simulink model "Quadrotor"  (Simulink 10.2)
settings: Solver=ode1  StartTime=0.0  StopTime=10  FixedStep=1e-4  RelTol=1e-3
settings Model: Creator=贺嘉辣  LastModifiedBy=贺嘉辣
settings DataIOCC: SaveFormat=Dataset  SignalLoggingSaveFormat=Dataset  ReturnWorkspaceOutputs=on
settings OptimizationCC: LifeSpan=auto
settings DebuggingCC: UnderspecifiedInitializationDetection=Simplified  MergeDetectMultiDrivingBlocksExec=error  FcnCallInpInsideContextMsg=error  SFUnexpectedBacktrackingDiag=error  SFNoUnconditionalDefaultTransitionDiag=error  SFExecutionAtInitializationDiag=warning  ArithmeticOperatorsInVariantConditions=error
settings HardwareCC: ProdBitPerPointer=64  ProdBitPerSizeT=64  ProdBitPerPtrDiffT=64  ProdLargestAtomicFloat=Float  ProdIntDivRoundTo=Zero  ProdEndianess=LittleEndian  ProdWordSize=64  ProdHWDeviceType=Intel->x86-64 (Windows64)
settings ModelReferenceCC: PropagateSignalLabelsOutOfModel=on
settings SFSimCC: SimUseLocalCustomCode=on  CustomCodeUndefinedFunction=FilterOut
settings RTWCC: RTWUseLocalCustomCode=on
settings CodeAppCC: StateflowObjectComments=off
settings GRTTargetCC: TargetLangStandard=C99 (ISO)  CombineOutputUpdateFcns=on  GRTInterface=off
settings ConfigComp: CovMetricSettings=dwe  CovSaveCumulativeToWorkspaceVar=off  CovSaveSingleToWorkspaceVar=off  CovExternalEMLEnable=on

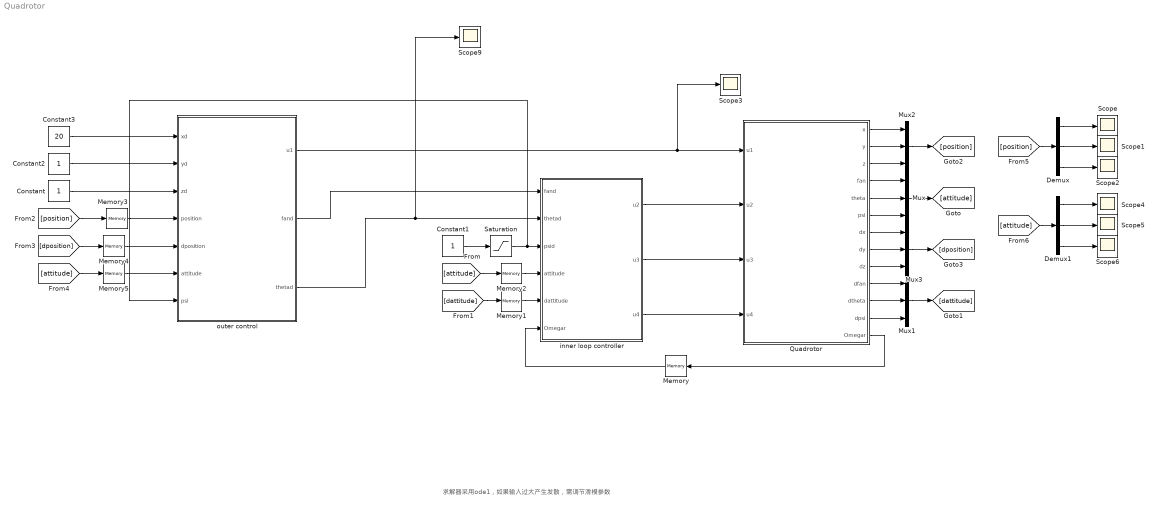
== system Quadrotor ==
  note: 求解器采用ode1，如果输入过大产生发散，需调节滑模参数
  Constant : Constant
  Constant1 : Constant
  Constant2 : Constant
  Constant3 : Constant  Value=20
  Demux : Demux  Outputs=3
  Demux1 : Demux  Outputs=3
  Memory{,1..5} (6 alike) : Memory
  Mux{,1..3} (4 alike) : Mux  Inputs=[1 1 1]
  Quadrotor : Subsystem  mask{m=0.65, g=9.8, Ixx=7.5e-3, Iyy=7.5e-3, Izz=1.3e-2, L=0.23, rho=3.1e-5, gama=7.5e-7, Ir=6e-5}
      mask prompts: m "无人机质量"; g "重力加速度"; Ixx "四旋翼绕X轴转动惯量"; Iyy "四旋翼绕Y轴转动惯量"; Izz "四旋翼绕Z轴转动惯量"; L "四旋翼臂长"; rho "四旋翼升力系数"; gama "空气阻力系数"; Ir "四旋翼转子转动惯量"
  Saturation : Saturate  UpperLimit=pi  LowerLimit=-pi
  Scope{,1..6,9} (8 alike) : Scope
  inner loop controller : Subsystem  mask{Ir=6e-5, Ixx=7.5e-3, Iyy=7.5e-3, Izz=1.3e-2}
      mask prompts: Ir "无人机转子惯量"; Ixx "无人机绕x轴转动惯量"; Iyy "无人机绕y轴转动惯量"; Izz "无人机绕z轴转动惯量"
  outer control : Subsystem  mask{m=0.65, g=9.8}
      mask prompts: m "无人机质量"; g "重力加速度"
  wires:
  inner loop controller/1(u2) -> Quadrotor/2(u2)
  inner loop controller/2(u3) -> Quadrotor/3(u3)
  Quadrotor/4(fan) -> Mux/1
  Quadrotor/5(theta) -> Mux/2
  Quadrotor/6(psi) -> Mux/3
  Mux/1 -> [attitude]
  Quadrotor/10(dfan) -> Mux1/1
  Quadrotor/11(dtheta) -> Mux1/2
  Quadrotor/12(dpsi) -> Mux1/3
  Mux1/1 -> [dattitude]
  [dattitude] -> Memory1/1
  [attitude] -> Memory2/1
  Quadrotor/13(Omegar) -> Memory/1
  Quadrotor/1(x) -> Mux2/1
  Quadrotor/2(y) -> Mux2/2
  Quadrotor/3(z) -> Mux2/3
  Mux2/1 -> [position]
  Memory/1 -> inner loop controller/6(Omegar)
  Memory1/1 -> inner loop controller/5(dattitude)
  Memory2/1 -> inner loop controller/4(attitude)
  Quadrotor/7(dx) -> Mux3/1
  Quadrotor/8(dy) -> Mux3/2
  Quadrotor/9(dz) -> Mux3/3
  Mux3/1 -> [dposition]
  [position] -> Memory3/1
  [dposition] -> Memory4/1
  Memory3/1 -> outer control/4(position)
  Memory4/1 -> outer control/5(dposition)
  [attitude] -> Memory5/1
  Memory5/1 -> outer control/6(attitude)
  Constant/1 -> outer control/3(zd)
  Constant1/1 -> Saturation/1
  Constant2/1 -> outer control/2(yd)
  Constant3/1 -> outer control/1(xd)
  inner loop controller/3(u4) -> Quadrotor/4(u4)
  outer control/2(fand) -> inner loop controller/1(fand)
  outer control/3(thetad) -> Scope9/1, inner loop controller/2(thetad)
  outer control/1(u1) -> Scope3/1, Quadrotor/1(u1)
  Saturation/1 -> outer control/7(psi), inner loop controller/3(psid)
  [position] -> Demux/1
  Demux/1 -> Scope/1
  Demux/2 -> Scope1/1
  Demux/3 -> Scope2/1
  [attitude] -> Demux1/1
  Demux1/3 -> Scope6/1
  Demux1/2 -> Scope5/1
  Demux1/1 -> Scope4/1

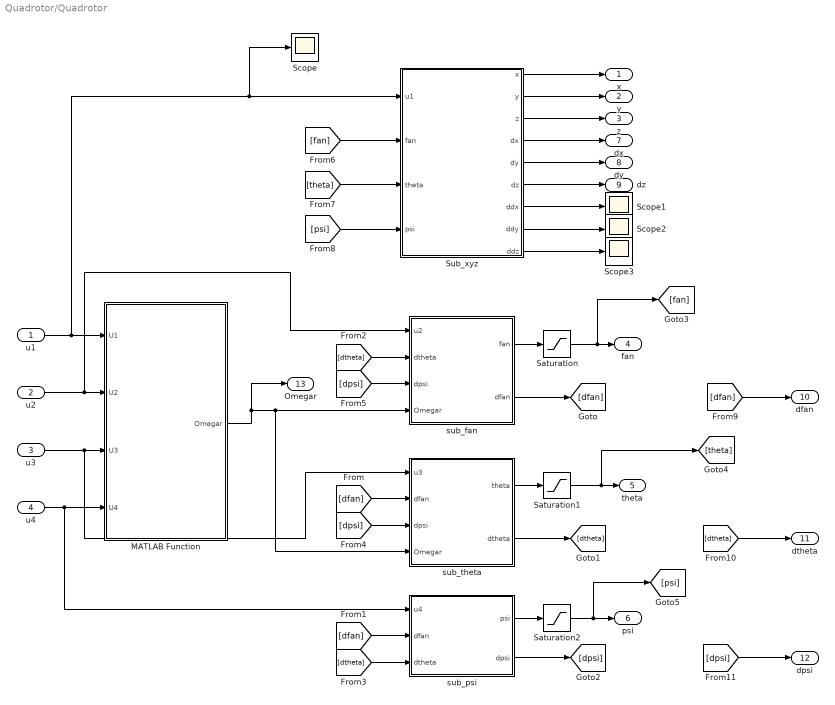
== system Quadrotor/Quadrotor ==
  u1 : Inport
  u2 : Inport  Port=2
  u3 : Inport  Port=3
  u4 : Inport  Port=4
  MATLAB Function : MATLAB Function  TreatAsAtomicUnit=on
  Saturation : Saturate  UpperLimit=pi/2  LowerLimit=-pi/2
  Saturation1 : Saturate  UpperLimit=pi/2  LowerLimit=-pi/2
  Saturation2 : Saturate  UpperLimit=pi  LowerLimit=-pi
  Scope{,1..3} (4 alike) : Scope
  Sub_xyz : Subsystem
  sub_fan : Subsystem
  sub_psi : Subsystem
  sub_theta : Subsystem
  x : Outport
  y : Outport  Port=2
  z : Outport  Port=3
  fan : Outport  Port=4
  theta : Outport  Port=5
  psi : Outport  Port=6
  dx : Outport  Port=7
  dy : Outport  Port=8
  dz : Outport  Port=9
  dfan : Outport  Port=10
  dtheta : Outport  Port=11
  dpsi : Outport  Port=12
  Omegar : Outport  Port=13
  wires:
  u2/1 -> sub_fan/1(u2), MATLAB Function/2(U2)
  u3/1 -> sub_theta/1(u3), MATLAB Function/3(U3)
  u4/1 -> sub_psi/1(u4), MATLAB Function/4(U4)
  sub_fan/1(fan) -> Saturation/1
  sub_theta/1(theta) -> Saturation1/1
  sub_psi/1(psi) -> Saturation2/1
  sub_fan/2(dfan) -> [dfan]
  [dfan] -> sub_theta/2(dfan)
  [dfan] -> sub_psi/2(dfan)
  sub_theta/2(dtheta) -> [dtheta]
  sub_psi/2(dpsi) -> [dpsi]
  [dtheta] -> sub_fan/2(dtheta)
  [dtheta] -> sub_psi/3(dtheta)
  [dpsi] -> sub_theta/3(dpsi)
  [dpsi] -> sub_fan/3(dpsi)
  u1/1 -> Scope/1, Sub_xyz/1(u1), MATLAB Function/1(U1)
  Sub_xyz/1(x) -> x/1
  Sub_xyz/2(y) -> y/1
  Sub_xyz/3(z) -> z/1
  [fan] -> Sub_xyz/2(fan)
  [theta] -> Sub_xyz/3(theta)
  [psi] -> Sub_xyz/4(psi)
  MATLAB Function/1(Omegar) -> Omegar/1, sub_theta/4(Omegar), sub_fan/4(Omegar)
  Sub_xyz/4(dx) -> dx/1
  Sub_xyz/5(dy) -> dy/1
  Sub_xyz/6(dz) -> dz/1
  [dfan] -> dfan/1
  [dtheta] -> dtheta/1
  [dpsi] -> dpsi/1
  Saturation/1 -> fan/1, [fan]
  Saturation1/1 -> theta/1, [theta]
  Saturation2/1 -> psi/1, [psi]
  Sub_xyz/7(ddx) -> Scope1/1
  Sub_xyz/8(ddy) -> Scope2/1
  Sub_xyz/9(ddz) -> Scope3/1

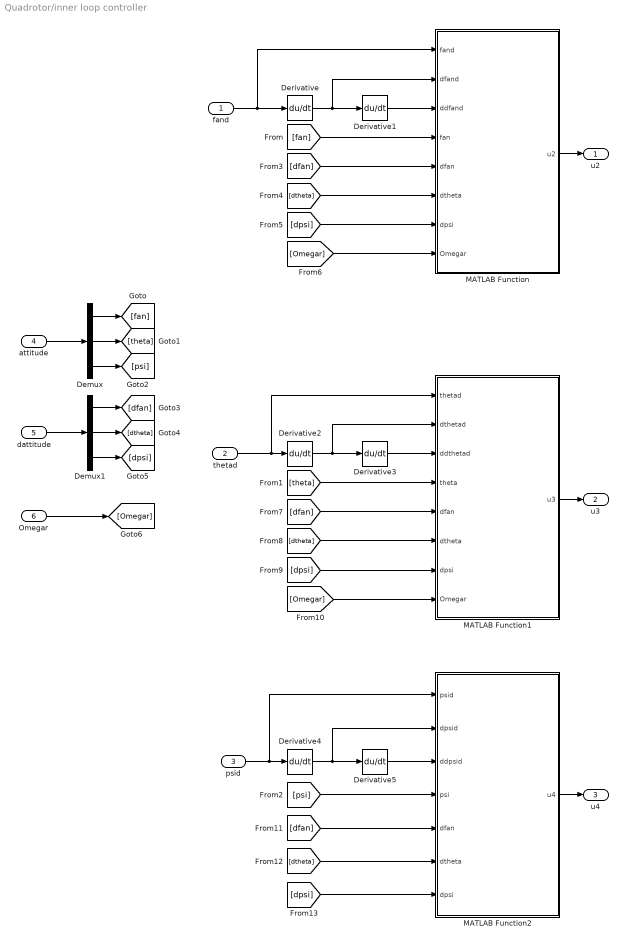
== system Quadrotor/inner loop controller ==
  fand : Inport
  thetad : Inport  Port=2
  psid : Inport  Port=3
  attitude : Inport  Port=4
  dattitude : Inport  Port=5
  Omegar : Inport  Port=6
  Demux : Demux  Outputs=[1 1 1]
  Demux1 : Demux  Outputs=[1 1 1]
  Derivative{,1..5} (6 alike) : Derivative
  MATLAB Function : MATLAB Function  TreatAsAtomicUnit=on
  MATLAB Function1 : MATLAB Function  TreatAsAtomicUnit=on
  MATLAB Function2 : MATLAB Function  TreatAsAtomicUnit=on
  u2 : Outport
  u3 : Outport  Port=2
  u4 : Outport  Port=3
  wires:
  fand/1 -> MATLAB Function/1(fand), Derivative/1
  Derivative/1 -> MATLAB Function/2(dfand), Derivative1/1
  Derivative1/1 -> MATLAB Function/3(ddfand)
  MATLAB Function/1(u2) -> u2/1
  attitude/1 -> Demux/1
  Demux/1 -> [fan]
  Demux/2 -> [theta]
  Demux/3 -> [psi]
  [fan] -> MATLAB Function/4(fan)
  dattitude/1 -> Demux1/1
  Demux1/3 -> [dpsi]
  Demux1/2 -> [dtheta]
  Demux1/1 -> [dfan]
  [dfan] -> MATLAB Function/5(dfan)
  [dtheta] -> MATLAB Function/6(dtheta)
  [dpsi] -> MATLAB Function/7(dpsi)
  Omegar/1 -> [Omegar]
  [Omegar] -> MATLAB Function/8(Omegar)
  Derivative2/1 -> MATLAB Function1/2(dthetad), Derivative3/1
  thetad/1 -> MATLAB Function1/1(thetad), Derivative2/1
  Derivative3/1 -> MATLAB Function1/3(ddthetad)
  MATLAB Function1/1(u3) -> u3/1
  [theta] -> MATLAB Function1/4(theta)
  [dfan] -> MATLAB Function1/5(dfan)
  [dtheta] -> MATLAB Function1/6(dtheta)
  [dpsi] -> MATLAB Function1/7(dpsi)
  [Omegar] -> MATLAB Function1/8(Omegar)
  Derivative4/1 -> MATLAB Function2/2(dpsid), Derivative5/1
  Derivative5/1 -> MATLAB Function2/3(ddpsid)
  psid/1 -> MATLAB Function2/1(psid), Derivative4/1
  [psi] -> MATLAB Function2/4(psi)
  [dpsi] -> MATLAB Function2/7(dpsi)
  [dtheta] -> MATLAB Function2/6(dtheta)
  [dfan] -> MATLAB Function2/5(dfan)
  MATLAB Function2/1(u4) -> u4/1

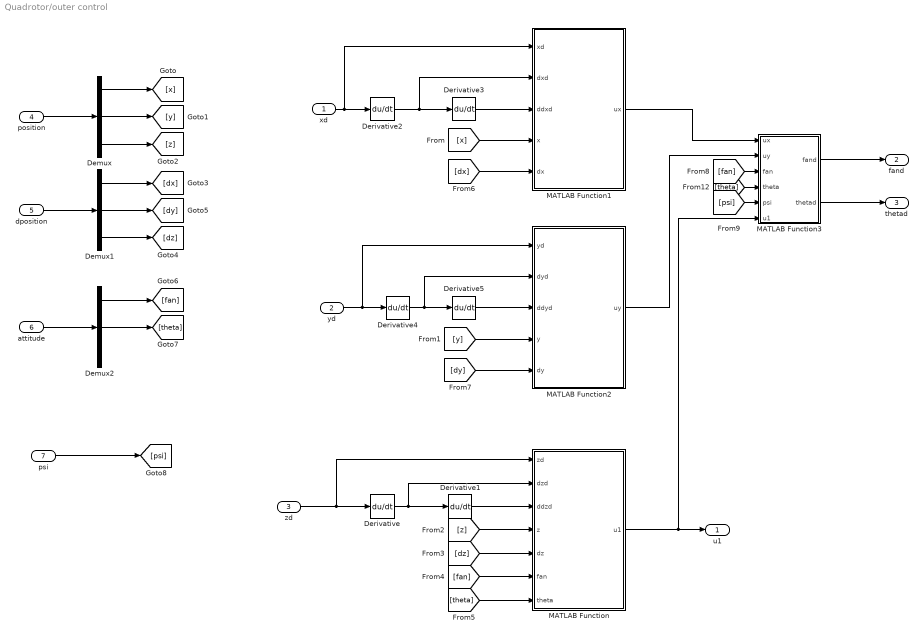
== system Quadrotor/outer control ==
  xd : Inport
  yd : Inport  Port=2
  zd : Inport  Port=3
  position : Inport  Port=4
  dposition : Inport  Port=5
  attitude : Inport  Port=6
  psi : Inport  Port=7
  Demux : Demux  Outputs=[1 1 1]
  Demux1 : Demux  Outputs=[1 1 1]
  Demux2 : Demux  Outputs=[1 1 1]
  Derivative{,1..5} (6 alike) : Derivative
  MATLAB Function : MATLAB Function  TreatAsAtomicUnit=on
  MATLAB Function1 : MATLAB Function  TreatAsAtomicUnit=on
  MATLAB Function2 : MATLAB Function  TreatAsAtomicUnit=on
  MATLAB Function3 : MATLAB Function  TreatAsAtomicUnit=on
  u1 : Outport
  fand : Outport  Port=2
  thetad : Outport  Port=3
  wires:
  zd/1 -> MATLAB Function/1(zd), Derivative/1
  Derivative/1 -> MATLAB Function/2(dzd), Derivative1/1
  position/1 -> Demux/1
  dposition/1 -> Demux1/1
  Demux/1 -> [x]
  Demux/2 -> [y]
  Demux/3 -> [z]
  Demux1/1 -> [dx]
  Demux1/3 -> [dz]
  Demux1/2 -> [dy]
  [z] -> MATLAB Function/4(z)
  [dz] -> MATLAB Function/5(dz)
  attitude/1 -> Demux2/1
  Demux2/1 -> [fan]
  Demux2/2 -> [theta]
  [fan] -> MATLAB Function/6(fan)
  [theta] -> MATLAB Function/7(theta)
  MATLAB Function/1(u1) -> MATLAB Function3/6(u1), u1/1
  Derivative2/1 -> MATLAB Function1/2(dxd), Derivative3/1
  xd/1 -> MATLAB Function1/1(xd), Derivative2/1
  [x] -> MATLAB Function1/4(x)
  [dx] -> MATLAB Function1/5(dx)
  yd/1 -> MATLAB Function2/1(yd), Derivative4/1
  Derivative4/1 -> MATLAB Function2/2(dyd), Derivative5/1
  [dy] -> MATLAB Function2/5(dy)
  [y] -> MATLAB Function2/4(y)
  MATLAB Function1/1(ux) -> MATLAB Function3/1(ux)
  MATLAB Function2/1(uy) -> MATLAB Function3/2(uy)
  [psi] -> MATLAB Function3/5(psi)
  MATLAB Function3/1(fand) -> fand/1
  MATLAB Function3/2(thetad) -> thetad/1
  [theta] -> MATLAB Function3/4(theta)
  [fan] -> MATLAB Function3/3(fan)
  Derivative3/1 -> MATLAB Function1/3(ddxd)
  Derivative5/1 -> MATLAB Function2/3(ddyd)
  Derivative1/1 -> MATLAB Function/3(ddzd)
  psi/1 -> [psi]

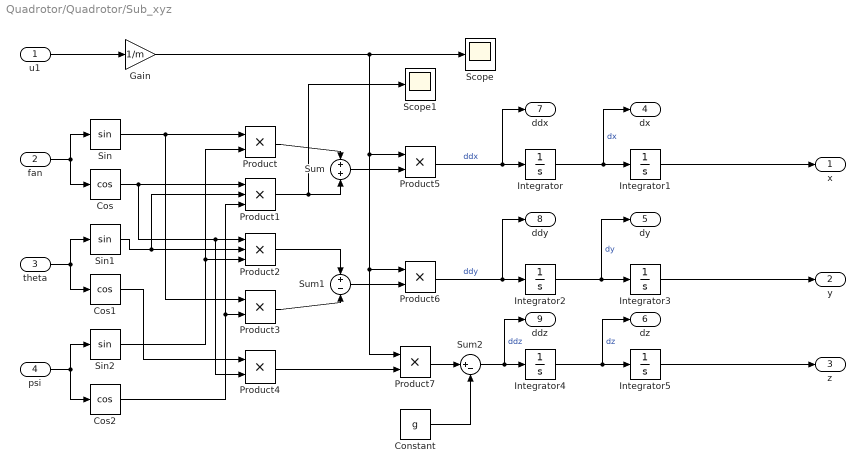
== system Quadrotor/Quadrotor/Sub_xyz ==
  u1 : Inport
  fan : Inport  Port=2
  theta : Inport  Port=3
  psi : Inport  Port=4
  Constant : Constant  Value=g
  Cos : Trigonometry  Operator=cos
  Cos1 : Trigonometry  Operator=cos
  Cos2 : Trigonometry  Operator=cos
  Gain : Gain  Gain=1/m
  Integrator{,1..5} (6 alike) : Integrator
  Product{,3..7} (6 alike) : Product
  Product1 : Product  Inputs=3
  Product2 : Product  Inputs=3
  Scope : Scope
  Scope1 : Scope
  Sin : Trigonometry
  Sin1 : Trigonometry
  Sin2 : Trigonometry
  Sum : Sum  Inputs=+|+
  Sum1 : Sum  Inputs=+|-
  Sum2 : Sum  Inputs=|+-
  x : Outport
  y : Outport  Port=2
  z : Outport  Port=3
  dx : Outport  Port=4
  dy : Outport  Port=5
  dz : Outport  Port=6
  ddx : Outport  Port=7
  ddy : Outport  Port=8
  ddz : Outport  Port=9
  wires:
  u1/1 -> Gain/1
  fan/1 -> Cos/1, Sin/1
  theta/1 -> Cos1/1, Sin1/1
  psi/1 -> Cos2/1, Sin2/1
  Sin/1 -> Product3/1, Product/1
  Sin2/1 -> Product/2, Product2/3
  Cos/1 -> Product4/2, Product2/1, Product1/1
  Sin1/1 -> Product2/2, Product1/2
  Cos2/1 -> Product1/3, Product3/2
  Product/1 -> Sum/1
  Product1/1 -> Scope1/1, Sum/2
  Cos1/1 -> Product4/1
  Product2/1 -> Sum1/1
  Product3/1 -> Sum1/2
  Sum/1 -> Product5/2
  Sum1/1 -> Product6/2
  Product4/1 -> Product7/2
  Gain/1 -> Scope/1, Product7/1, Product6/1, Product5/1
  Product5/1 -> ddx/1, Integrator/1  "ddx"
  Integrator/1 -> dx/1, Integrator1/1  "dx"
  Product6/1 -> ddy/1, Integrator2/1  "ddy"
  Integrator2/1 -> dy/1, Integrator3/1  "dy"
  Product7/1 -> Sum2/1
  Constant/1 -> Sum2/2
  Sum2/1 -> ddz/1, Integrator4/1  "ddz"
  Integrator4/1 -> dz/1, Integrator5/1  "dz"
  Integrator3/1 -> y/1
  Integrator1/1 -> x/1
  Integrator5/1 -> z/1

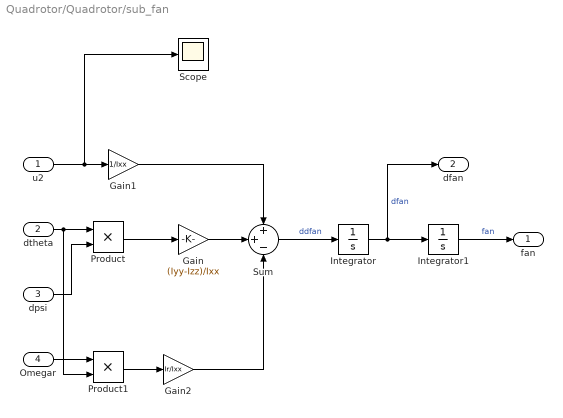
== system Quadrotor/Quadrotor/sub_fan ==
  u2 : Inport
  dtheta : Inport  Port=2
  dpsi : Inport  Port=3
  Omegar : Inport  Port=4
  Gain : Gain  Gain=(Iyy-Izz)/Ixx
  Gain1 : Gain  Gain=1/Ixx
  Gain2 : Gain  Gain=Ir/Ixx
  Integrator : Integrator
  Integrator1 : Integrator
  Product : Product
  Product1 : Product
  Scope : Scope
  Sum : Sum  Inputs=++-
  fan : Outport
  dfan : Outport  Port=2
  wires:
  Sum/1 -> Integrator/1  "ddfan"
  Integrator/1 -> dfan/1, Integrator1/1  "dfan"
  Integrator1/1 -> fan/1  "fan"
  dtheta/1 -> Product1/2, Product/1
  dpsi/1 -> Product/2
  Product/1 -> Gain/1
  Gain/1 -> Sum/2
  u2/1 -> Scope/1, Gain1/1
  Gain1/1 -> Sum/1
  Omegar/1 -> Product1/1
  Product1/1 -> Gain2/1
  Gain2/1 -> Sum/3

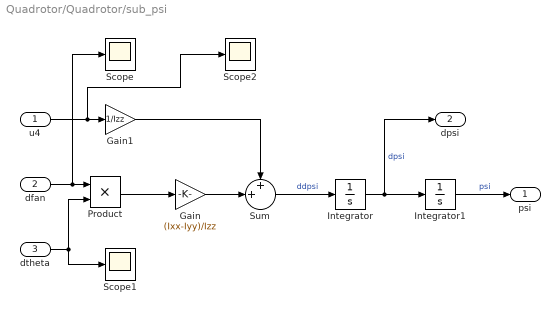
== system Quadrotor/Quadrotor/sub_psi ==
  u4 : Inport
  dfan : Inport  Port=2
  dtheta : Inport  Port=3
  Gain : Gain  Gain=(Ixx-Iyy)/Izz
  Gain1 : Gain  Gain=1/Izz
  Integrator : Integrator
  Integrator1 : Integrator
  Product : Product
  Scope : Scope
  Scope1 : Scope
  Scope2 : Scope
  Sum : Sum  Inputs=++|
  psi : Outport
  dpsi : Outport  Port=2
  wires:
  Sum/1 -> Integrator/1  "ddpsi"
  Integrator/1 -> dpsi/1, Integrator1/1  "dpsi"
  Integrator1/1 -> psi/1  "psi"
  dfan/1 -> Scope/1, Product/1
  dtheta/1 -> Scope1/1, Product/2
  Product/1 -> Gain/1
  Gain/1 -> Sum/2
  u4/1 -> Scope2/1, Gain1/1
  Gain1/1 -> Sum/1

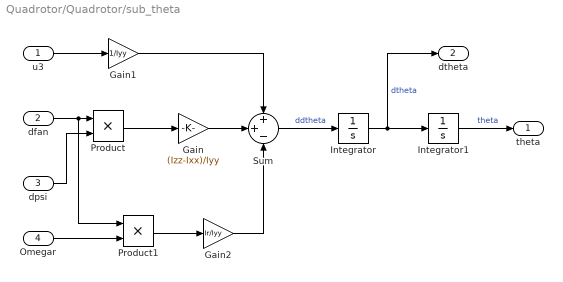
== system Quadrotor/Quadrotor/sub_theta ==
  u3 : Inport
  dfan : Inport  Port=2
  dpsi : Inport  Port=3
  Omegar : Inport  Port=4
  Gain : Gain  Gain=(Izz-Ixx)/Iyy
  Gain1 : Gain  Gain=1/Iyy
  Gain2 : Gain  Gain=Ir/Iyy
  Integrator : Integrator
  Integrator1 : Integrator
  Product : Product
  Product1 : Product
  Sum : Sum  Inputs=++-
  theta : Outport
  dtheta : Outport  Port=2
  wires:
  Sum/1 -> Integrator/1  "ddtheta"
  Integrator/1 -> dtheta/1, Integrator1/1  "dtheta"
  Integrator1/1 -> theta/1  "theta"
  dfan/1 -> Product1/1, Product/1
  dpsi/1 -> Product/2
  Product/1 -> Gain/1
  Gain/1 -> Sum/2
  u3/1 -> Gain1/1
  Gain1/1 -> Sum/1
  Omegar/1 -> Product1/2
  Product1/1 -> Gain2/1
  Gain2/1 -> Sum/3

== matlab function inner loop controller/MATLAB Function ==
  data: u2 output double; fand input double; dfand input double; ddfand input double; fan input double; dfan input double; dtheta input double; dpsi input double; Omegar input double; Ixx parameter double; Iyy parameter double; Izz parameter double; Ir parameter double
function u2 = fcn(fand, dfand, ddfand, fan, dfan, dtheta, dpsi, Omegar, Ixx, Iyy, Izz, Ir)
e = fan -fand;
de = dfan - dfand;
s = e + de;
f = dtheta*dpsi*(Iyy-Izz)/Ixx-Ir*dtheta*Omegar/Ixx;
u2 = Ixx*(ddfand+dfand-f-dfan-100*s-10*sat(s));

== matlab function Quadrotor/MATLAB Function ==
  data: U1 input double; Omegar output double; U2 input double; U3 input double; U4 input double; rho parameter double; L parameter double; gama parameter double
function Omegar = fcn(U1, U2, U3, U4, rho, L, gama)
%rho无人机升力系数 
%L四旋翼臂长
%gama无人机阻力系数
% rho = 3.1e-5;
% L = 0.23;
% gama = 7.5e-7;
B = [rho rho rho rho;
    0 -L*rho 0 L*rho;
    L*rho 0 -L*rho 0;
    -gama gama -gama gama];
U = [U1 U2 U3 U4]';
BU = B\U;
Omega1 = sqrt(abs(BU(1)));
Omega2 = sqrt(abs(BU(2)));
Omega3 = sqrt(abs(BU(3)));
Omega4 = sqrt(abs(BU(4)));
Omegar  = Omega1 - Omega2 + Omega3 - Omega4;

== matlab function inner loop controller/MATLAB Function1 ==
  data: u3 output double; thetad input double; dthetad input double; ddthetad input double; theta input double; dfan input double; dtheta input double; dpsi input double; Omegar input double; Ixx parameter double; Iyy parameter double; Izz parameter double; Ir parameter double
function u3 = fcn(thetad, dthetad, ddthetad, theta, dfan, dtheta, dpsi, Omegar, Ixx, Iyy, Izz, Ir)
e = theta -thetad;
de = dtheta - dthetad;
s = e + de;
f = dfan*dpsi*(Izz-Ixx)/Iyy-Ir*dfan*Omegar/Iyy;
u3 = Iyy*(ddthetad-f-de-100*s-10*sat(s));

== matlab function inner loop controller/MATLAB Function2 ==
  data: u4 output double; psid input double; dpsid input double; ddpsid input double; psi input double; dfan input double; dtheta input double; Ixx parameter double; Iyy parameter double; Izz parameter double; dpsi input double
function u4 = fcn(psid, dpsid, ddpsid, psi, dfan, dtheta, Ixx, Iyy, Izz, dpsi)
e = psi -psid;
de = dpsi - dpsid;
s = e + de;
f = dfan*dtheta*(Ixx-Iyy)/Izz;
u4 = Izz*(ddpsid-f-de-100*s-10*sat(s));

== matlab function outer control/MATLAB Function ==
  data: zd input double; u1 output double; dzd input double; ddzd input double; z input double; dz input double; fan input double; theta input double; m parameter double; g parameter double
function u1 = fcn(zd, dzd, ddzd, z, dz, fan, theta, m, g)
ez = z - zd;
dez = dz - dzd;
sz = ez + dez;
u1 = m*(g+ddzd-dez-5*sz-10*sat(sz))/(cos(theta)*cos(fan));

== matlab function outer control/MATLAB Function1 ==
  data: xd input double; ux output double; dxd input double; ddxd input double; x input double; dx input double; m parameter double
function ux = fcn(xd, dxd, ddxd, x, dx, m)
ex = x - xd;
dex = dx - dxd;
sx = ex + dex;
%滑模
ux = m*(ddxd-dex-sx-5*sat(sx));
%反演
% z1 = x - xd;
% dz1 = dx - dxd;
% alpha = dxd - 0.5*z1;
% dalpha = ddxd - 0.5*dz1;
% z2 = dx - alpha;
% ux = m*(dalpha-z1-0.5*z2);

== matlab function outer control/MATLAB Function2 ==
  data: yd input double; uy output double; dyd input double; ddyd input double; y input double; dy input double; m parameter double
function uy = fcn(yd, dyd, ddyd, y, dy, m)
ey = y - yd;
dey = dy - dyd;
sy = ey + dey;
uy = m*(ddyd-dey-sy-5*sat(sy));

% z1 = y - yd;
% dz1 = dy - dyd;
% alpha = dyd - z1;
% dalpha = ddyd - dz1;
% z2 = dy - alpha;
% uy = m*(dalpha-z1-z2);

== matlab function outer control/MATLAB Function3 ==
  data: ux input double; fand output double; uy input double; fan input double; theta input double; psi input double; thetad output double; u1 input double
function [fand, thetad] = fcn(ux, uy, fan, theta, psi, u1)

k1 = (ux*sin(psi)-uy*cos(psi))/u1;
% k2 = (ux*cos(psi)+uy*sin(psi))/(cos(theta)*cos(fan)*u1);
k2 = (ux-sin(fan)*sin(psi))/(cos(fan)*cos(psi)*u1);
if k1>=0.9
    k1 = 0.9;
elseif k1<=-0.9
    k1 = -0.9;    
end

if k2>=0.9
    k2 = 0.9;
elseif k2<=-0.9
    k2 = -0.9;    
end
fand = asin(k1);
thetad = asin(k2);
%thetad = atan(k2);
